simulink model "SWC_FDC_type"  (R2021b)
settings: Solver=FixedStepDiscrete  StartTime=0.0  StopTime=10.0  FixedStep=0.001  RelTol=1e-3
values from neighbouring files (symbols this model uses):
  C_TASK_5MS_S = (	C_TICK_TIME_S      	)    [vcu_local_hdr.m]
  DID_VCUKey = uint16(0x0202)    [vcu_local_hdr.m]
  DID_XWD = uint16(513)    [vcu_local_hdr.m]
  DIDLen_APPPedalZP = uint16(3)    [vcu_local_hdr.m]
  DIDLen_APSFunConfig = uint16(16)    [vcu_local_hdr.m]
  DIDLen_AutoLock = uint16(1)    [vcu_local_hdr.m]
  DIDLen_AutoWipHSpdEN = uint16(1)    [vcu_local_hdr.m]
  DIDLen_DKCKey = uint16(8)    [vcu_local_hdr.m]
  DIDLen_DRLDis = uint16(1)    [vcu_local_hdr.m]
  DIDLen_DynoMode = uint16(1)    [vcu_local_hdr.m]
  DIDLen_FMHTimer = uint16(1)    [vcu_local_hdr.m]
  DIDLen_LFLowPresThre = uint16(1)    [vcu_local_hdr.m]
  DIDLen_LFSensorID = uint16(4)    [vcu_local_hdr.m]
  DIDLen_LRLowPresThre = uint16(1)    [vcu_local_hdr.m]
  DIDLen_LRSensorID = uint16(4)    [vcu_local_hdr.m]
  DIDLen_NVMPedalZP = uint16(3)    [vcu_local_hdr.m]
  DIDLen_RFLowPresThre = uint16(1)    [vcu_local_hdr.m]
  DIDLen_RFSensorID = uint16(4)    [vcu_local_hdr.m]
  DIDLen_RRLowPresThre = uint16(1)    [vcu_local_hdr.m]
  DIDLen_RRSensorID = uint16(4)    [vcu_local_hdr.m]
  DIDLen_SensorMode = uint16(1)    [vcu_local_hdr.m]
  DIDLen_TireSize = uint16(16)    [vcu_local_hdr.m]
  DIDLen_TPMSLearnSta = uint16(1)    [vcu_local_hdr.m]
  DIDLen_TurnLampFLThreCurr = uint16(1)    [vcu_local_hdr.m]
  DIDLen_TurnLampFRThreCurr = uint16(1)    [vcu_local_hdr.m]
  DIDLen_TurnLampRLThreCurr = uint16(1)    [vcu_local_hdr.m]
  DIDLen_TurnLampRRThreCurr = uint16(1)    [vcu_local_hdr.m]
  DIDLen_USSConfig = uint16(16)    [vcu_local_hdr.m]
  DIDLen_WhlPres = uint16(4)    [vcu_local_hdr.m]
  DIDLen_WhlSensorBattSta = uint16(1)    [vcu_local_hdr.m]
  DIDLen_WhlTmp = uint16(4)    [vcu_local_hdr.m]
  DIDLen_WipRLSCmdCutFilter = uint16(1)    [vcu_local_hdr.m]
  DIDLen_WipRLSCmdHoldFilter = uint16(1)    [vcu_local_hdr.m]
  DIDLen_XWDMode = uint16(1)    [vcu_local_hdr.m]
  DIDNum_APPPedalZP = uint16(0x0206)    [vcu_local_hdr.m]
  DIDNum_APSFunConfig = uint16(0x0903)    [vcu_local_hdr.m]
  DIDNum_AutoLock = uint16(0x0306)    [vcu_local_hdr.m]
  DIDNum_AutoWipHSpdEN = uint16(0x0308)    [vcu_local_hdr.m]
  DIDNum_DKCKey = uint16(0x0202)    [vcu_local_hdr.m]
  DIDNum_DRLDis = uint16(0x0307)    [vcu_local_hdr.m]
  DIDNum_DynoMode = uint16(0x0203)    [vcu_local_hdr.m]
  DIDNum_FMHTimer = uint16(0x0305)    [vcu_local_hdr.m]
  DIDNum_LFLowPresThre = uint16(0x0B08)    [vcu_local_hdr.m]
  DIDNum_LFSensorID = uint16(0x0B01)    [vcu_local_hdr.m]
  DIDNum_LRLowPresThre = uint16(0x0B0A)    [vcu_local_hdr.m]
  DIDNum_LRSensorID = uint16(0x0B03)    [vcu_local_hdr.m]
  DIDNum_NVMPedalZP = uint16(0x0207)    [vcu_local_hdr.m]
  DIDNum_RFLowPresThre = uint16(0x0B09)    [vcu_local_hdr.m]
  DIDNum_RFSensorID = uint16(0x0B02)    [vcu_local_hdr.m]
  DIDNum_RRLowPresThre = uint16(0x0B0B)    [vcu_local_hdr.m]
  DIDNum_RRSensorID = uint16(0x0B04)    [vcu_local_hdr.m]
  DIDNum_SensorMode = uint16(0x0B0C)    [vcu_local_hdr.m]
  DIDNum_TireSize = uint16(0x0902)    [vcu_local_hdr.m]
  DIDNum_TPMSLearnSta = uint16(0x0B0D)    [vcu_local_hdr.m]
  DIDNum_TurnLampFLThreCurr = uint16(0x0303)    [vcu_local_hdr.m]
  DIDNum_TurnLampFRThreCurr = uint16(0x0301)    [vcu_local_hdr.m]
  DIDNum_TurnLampRLThreCurr = uint16(0x0304)    [vcu_local_hdr.m]
  DIDNum_TurnLampRRThreCurr = uint16(0x0302)    [vcu_local_hdr.m]
  DIDNum_USSConfig = uint16(0x0901)    [vcu_local_hdr.m]
  DIDNum_WhlPres = uint16(0x0B05)    [vcu_local_hdr.m]
  DIDNum_WhlSensorBattSta = uint16(0x0B07)    [vcu_local_hdr.m]
  DIDNum_WhlTmp = uint16(0x0B06)    [vcu_local_hdr.m]
  DIDNum_WipRLSCmdCutFilter = uint16(0x030A)    [vcu_local_hdr.m]
  DIDNum_WipRLSCmdHoldFilter = uint16(0x0309)    [vcu_local_hdr.m]
  DIDNum_XWDMode = uint16(0x0201)    [vcu_local_hdr.m]
  DIDVCUKeyLength = uint16(8)    [vcu_local_hdr.m]
  DTC_10020B = Simulink.Parameter    [DTC_Constant_Definition.m]
  DTC_10020C = Simulink.Parameter    [DTC_Constant_Definition.m]
  DTC_10020D = Simulink.Parameter    [DTC_Constant_Definition.m]
  DTC_10020E = Simulink.Parameter    [DTC_Constant_Definition.m]
  DTC_100210 = Simulink.Parameter    [DTC_Constant_Definition.m]
  DTC_100211 = Simulink.Parameter    [DTC_Constant_Definition.m]
  DTC_100212 = Simulink.Parameter    [DTC_Constant_Definition.m]
  DTC_100213 = Simulink.Parameter    [DTC_Constant_Definition.m]
  DTC_100214 = Simulink.Parameter    [DTC_Constant_Definition.m]
  DTC_100215 = Simulink.Parameter    [DTC_Constant_Definition.m]
  DTC_100216 = Simulink.Parameter    [DTC_Constant_Definition.m]
  DTC_100217 = Simulink.Parameter    [DTC_Constant_Definition.m]
  DTC_100218 = Simulink.Parameter    [DTC_Constant_Definition.m]
  DTC_100219 = Simulink.Parameter    [DTC_Constant_Definition.m]
  DTC_10021A = Simulink.Parameter    [DTC_Constant_Definition.m]
  DTC_10021B = Simulink.Parameter    [DTC_Constant_Definition.m]
  DTC_10021C = Simulink.Parameter    [DTC_Constant_Definition.m]
  DTC_10021D = Simulink.Parameter    [DTC_Constant_Definition.m]
  DTC_10021E = Simulink.Parameter    [DTC_Constant_Definition.m]
  DTC_100220 = Simulink.Parameter    [DTC_Constant_Definition.m]
  DTC_100221 = Simulink.Parameter    [DTC_Constant_Definition.m]
  DTC_100223 = Simulink.Parameter    [DTC_Constant_Definition.m]
  DTC_100224 = Simulink.Parameter    [DTC_Constant_Definition.m]
  DTC_100225 = Simulink.Parameter    [DTC_Constant_Definition.m]
  DTC_100226 = Simulink.Parameter    [DTC_Constant_Definition.m]
  DTC_100227 = Simulink.Parameter    [DTC_Constant_Definition.m]
  DTC_100242 = Simulink.Parameter    [DTC_Constant_Definition.m]
  DTC_100243 = Simulink.Parameter    [DTC_Constant_Definition.m]
  DTC_100244 = Simulink.Parameter    [DTC_Constant_Definition.m]
  DTC_100247 = Simulink.Parameter    [DTC_Constant_Definition.m]
  DTC_100248 = Simulink.Parameter    [DTC_Constant_Definition.m]
  DTC_100249 = Simulink.Parameter    [DTC_Constant_Definition.m]
  DTC_100250 = Simulink.Parameter    [DTC_Constant_Definition.m]
  DTC_100251 = Simulink.Parameter    [DTC_Constant_Definition.m]
  DTC_100252 = Simulink.Parameter    [DTC_Constant_Definition.m]
  DTC_100A10 = Simulink.Parameter    [DTC_Constant_Definition.m]
  DTC_100A12 = Simulink.Parameter    [DTC_Constant_Definition.m]
  DTC_100A16 = Simulink.Parameter    [DTC_Constant_Definition.m]
  DTC_100A17 = Simulink.Parameter    [DTC_Constant_Definition.m]
  DTC_100A18 = Simulink.Parameter    [DTC_Constant_Definition.m]
  DTC_100A19 = Simulink.Parameter    [DTC_Constant_Definition.m]
  DTC_500B01 = Simulink.Parameter    [DTC_Constant_Definition.m]
  DTC_500B02 = Simulink.Parameter    [DTC_Constant_Definition.m]
  DTC_500B03 = Simulink.Parameter    [DTC_Constant_Definition.m]
  DTC_500B04 = Simulink.Parameter    [DTC_Constant_Definition.m]
  DTC_500B05 = Simulink.Parameter    [DTC_Constant_Definition.m]
  DTC_500B06 = Simulink.Parameter    [DTC_Constant_Definition.m]
  DTC_500B07 = Simulink.Parameter    [DTC_Constant_Definition.m]
  DTC_500B08 = Simulink.Parameter    [DTC_Constant_Definition.m]
  DTC_500B09 = Simulink.Parameter    [DTC_Constant_Definition.m]
  DTC_500B0A = Simulink.Parameter    [DTC_Constant_Definition.m]
  DTC_500B0B = Simulink.Parameter    [DTC_Constant_Definition.m]
  DTC_500B0C = Simulink.Parameter    [DTC_Constant_Definition.m]
  DTC_500B0D = Simulink.Parameter    [DTC_Constant_Definition.m]
  ... (+93 more)
undefined symbols (not defined in the file or in its folder): f32_ApsOutVehSpdSig, KHAL_CANBusOffDebounce_cnt, KHAL_CANBusOffDebounce_s, KHAL_DKCDecryptEnable_flg_ovrdflg, KHAL_DKCDecryptEnable_flg_ovrdval, KHAL_RandomNumberY1_enum, KHAL_RandomNumberY2_enum, KHAL_RandomNumberY_ovrdflg, KHAL_TPMSRESBUTT_flg_ovrdflg, KHAL_TPMSRESBUTT_flg_ovrdval, KINP_ReadVinCode_flg, KTQD_DefaultRegenMode_enum, R_DIDWriteCDD_CSOP_DIDSet_APPPedalZP, R_DIDWriteCDD_CSOP_DIDSet_APSFunConfig, R_DIDWriteCDD_CSOP_DIDSet_AutoLock, R_DIDWriteCDD_CSOP_DIDSet_AutoWipHSpdEN, R_DIDWriteCDD_CSOP_DIDSet_DKCKey, R_DIDWriteCDD_CSOP_DIDSet_DRLDis, R_DIDWriteCDD_CSOP_DIDSet_DynoMode, R_DIDWriteCDD_CSOP_DIDSet_FMHTimer, R_DIDWriteCDD_CSOP_DIDSet_LFLowPresThre, R_DIDWriteCDD_CSOP_DIDSet_LFSensorID, R_DIDWriteCDD_CSOP_DIDSet_LRLowPresThre, R_DIDWriteCDD_CSOP_DIDSet_LRSensorID, R_DIDWriteCDD_CSOP_DIDSet_NVMPedalZP, R_DIDWriteCDD_CSOP_DIDSet_RFLowPresThre, R_DIDWriteCDD_CSOP_DIDSet_RFSensorID, R_DIDWriteCDD_CSOP_DIDSet_RRLowPresThre, R_DIDWriteCDD_CSOP_DIDSet_RRSensorID, R_DIDWriteCDD_CSOP_DIDSet_SensorMode, R_DIDWriteCDD_CSOP_DIDSet_TireSize, R_DIDWriteCDD_CSOP_DIDSet_TPMSLearnSta, R_DIDWriteCDD_CSOP_DIDSet_TurnLampFLThreCurr, R_DIDWriteCDD_CSOP_DIDSet_TurnLampFRThreCurr, R_DIDWriteCDD_CSOP_DIDSet_TurnLampRLThreCurr, R_DIDWriteCDD_CSOP_DIDSet_TurnLampRRThreCurr, R_DIDWriteCDD_CSOP_DIDSet_USSConfig, R_DIDWriteCDD_CSOP_DIDSet_WhlPres, R_DIDWriteCDD_CSOP_DIDSet_WhlSensorBattSta, R_DIDWriteCDD_CSOP_DIDSet_WhlTmp, R_DIDWriteCDD_CSOP_DIDSet_WipRLSCmdCutFilter, R_DIDWriteCDD_CSOP_DIDSet_WipRLSCmdHoldFilter, R_DIDWriteCDD_CSOP_DIDSet_XWDMode, R_E2E_CAN3_VCU1_CSOP_Write_CAN3_VCU1, R_E2E_CAN3_VCU1_toNIDEC_CSOP_Write_CAN3_VCU1_toNIDEC ... (+128)
libraries: simulink x246, FVT_lib x139, hcu_lib x31, hdlsllib x11, app x1, halin x1, halout x1, matrix_library x1, inp x1, outp x1
(part 5 of 13)

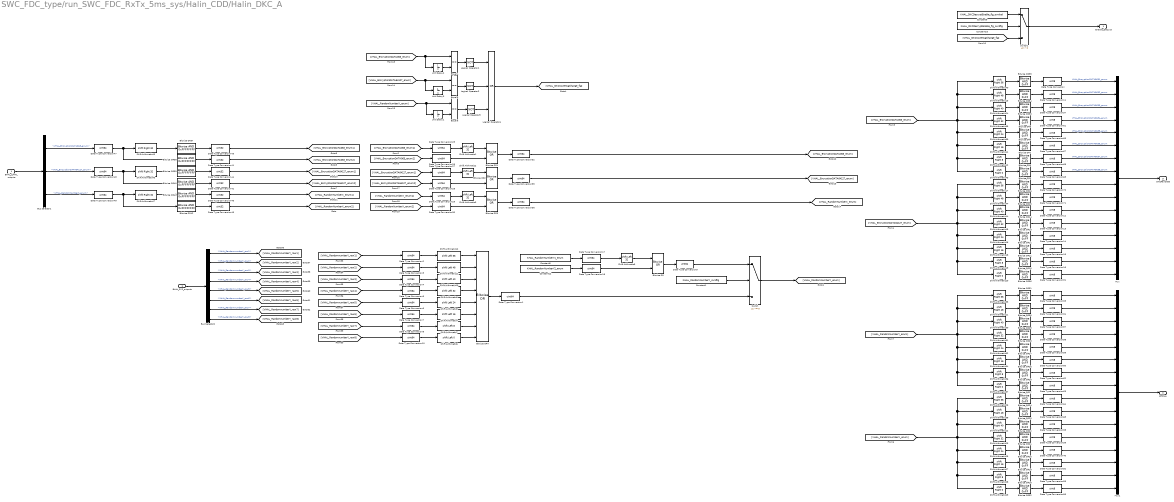
== system SWC_FDC_type/run_SWC_FDC_RxTx_5ms_sys/Halin_CDD/Halin_DKC_A ==
  BHAL_CAN4_outputs : Inport
  BHAL_SYS_outputs : Inport  Port=2
  Bitwise OR{,1..3} (4 alike) : simulink/Logic and Bit Operations/Bitwise Operator  logicop=OR  UseBitMask=off  NumInputPorts=2  BitMask=bin2dec('11011001')  BitMaskRealWorld=Stored Integer
  Bitwise OR{5..36} (32 alike) : simulink/Logic and Bit Operations/Bitwise Operator  logicop=AND  UseBitMask=on  BitMask=0xFF  BitMaskRealWorld=Stored Integer
  Bitwise OR{37..42} (6 alike) : simulink/Logic and Bit Operations/Bitwise Operator  logicop=AND  UseBitMask=on  BitMask=0xFFFFFFFF  BitMaskRealWorld=Stored Integer
  Bitwise OR4 : simulink/Logic and Bit Operations/Bitwise Operator  logicop=OR  UseBitMask=off  NumInputPorts=8  BitMask=bin2dec('11011001')  BitMaskRealWorld=Stored Integer
  Bus Selector1 : BusSelector  OutputSignals=VHAL_EncryptionDATA063_enum,VHAL_EncryptionDATA64127_enum,VHAL_RandomNumberX_enum
  Bus Selector2 : BusSelector  OutputSignals=VHAL_RandomnumberY_raw1,VHAL_RandomnumberY_raw2,VHAL_RandomnumberY_raw3,VHAL_RandomnumberY_raw4,VHAL_RandomnumberY_raw5,VHAL_RandomnumberY_raw6,VHAL_RandomnumberY_raw7,VHAL_RandomnumberY_raw8
  Constant1 : Constant  Value=KHAL_RandomNumberY_ovrdflg  OutDataTypeStr=uint64
  Constant10 : Constant  Value=KHAL_DKCDecryptEnable_flg_ovrdflg
  Constant12 : Constant  Value=KHAL_RandomNumberY2_enum  OutDataTypeStr=uint64
  Constant5 : Constant  Value=KHAL_RandomNumberY1_enum  OutDataTypeStr=uint64
  Constant9 : Constant  Value=KHAL_DKCDecryptEnable_flg_ovrdval
  Data Type Conversion{,11..16,31,33..34,37..40,52,55..71} (32 alike) : DataTypeConversion  OutDataTypeStr=uint8
  Data Type Conversion{1..10,17..18,25..30,32,35..36,47..49} (24 alike) : DataTypeConversion  OutDataTypeStr=uint64
  Data Type Conversion{41..46} (6 alike) : DataTypeConversion  OutDataTypeStr=uint32
  Equal4 : RelationalOperator  Operator===  OutDataTypeStr=boolean  RndMeth=Simplest
  Equal5 : RelationalOperator  Operator===  OutDataTypeStr=boolean  RndMeth=Simplest
  Equal6 : RelationalOperator  Operator===  OutDataTypeStr=boolean  RndMeth=Simplest
  Logical Operator1 : Logic  Operator=NOT  AllPortsSameDT=off  OutDataTypeStr=boolean
  Logical Operator2 : Logic  Operator=NOT  AllPortsSameDT=off  OutDataTypeStr=boolean
  Logical Operator3 : Logic  Operator=NOT  AllPortsSameDT=off  OutDataTypeStr=boolean
  Logical Operator4 : Logic  Operator=OR  Inputs=3  AllPortsSameDT=off  OutDataTypeStr=boolean
  Mux : Mux  Inputs=16
  Mux1 : Mux  Inputs=16
  Shift Arithmetic{1..3,5,9} (5 alike) : ArithShift  BitShiftNumber=32  BitShiftDirection=Left
  Shift Arithmetic10 : ArithShift  BitShiftNumber=40  BitShiftDirection=Left
  Shift Arithmetic11 : ArithShift  BitShiftNumber=48  BitShiftDirection=Left
  Shift Arithmetic12 : ArithShift  BitShiftNumber=56  BitShiftDirection=Left
  Shift Arithmetic{13,21,38,44} (4 alike) : ArithShift  BitShiftNumber=48  BitShiftDirection=Right
  Shift Arithmetic{14,22,24,30} (4 alike) : ArithShift  BitShiftNumber=40  BitShiftDirection=Right
  Shift Arithmetic{15,23,31,35,45..47} (7 alike) : ArithShift  BitShiftNumber=32  BitShiftDirection=Right
  Shift Arithmetic{16,25,32,39} (4 alike) : ArithShift  BitShiftNumber=24  BitShiftDirection=Right
  Shift Arithmetic{17,26,33,40} (4 alike) : ArithShift  BitShiftNumber=56  BitShiftDirection=Right
  Shift Arithmetic{18,27,34,41} (4 alike) : ArithShift  BitShiftNumber=16  BitShiftDirection=Right
  Shift Arithmetic{19,28,36,42} (4 alike) : ArithShift  BitShiftNumber=8  BitShiftDirection=Right
  Shift Arithmetic{20,29,37,43} (4 alike) : ArithShift  BitShiftDirection=Right
  Shift Arithmetic4 : ArithShift  BitShiftNumber=16  BitShiftDirection=Left
  Shift Arithmetic6 : ArithShift  BitShiftDirection=Left
  Shift Arithmetic7 : ArithShift  BitShiftNumber=8  BitShiftDirection=Left
  Shift Arithmetic8 : ArithShift  BitShiftNumber=24  BitShiftDirection=Left
  Switch : Switch  Criteria=u2 ~= 0
  Switch1 : Switch  Criteria=u2 > Threshold
  Unit Delay1 : UnitDelay  SampleTime=-1  HasFrameUpgradeWarning=on
  Unit Delay2 : UnitDelay  SampleTime=-1  HasFrameUpgradeWarning=on
  Unit Delay3 : UnitDelay  SampleTime=-1  HasFrameUpgradeWarning=on
  Enable_Decrypt : Outport
  AESKey : Outport  Port=2
  DKCRawData : Outport  Port=3
  wires:
  Data Type Conversion8/1 -> Shift Arithmetic7/1
  Bitwise OR5/1 -> Data Type Conversion69/1
  [VHAL_RandomNumberX_enum] -> Shift Arithmetic38/1, Shift Arithmetic26/1, Shift Arithmetic22/1, Shift Arithmetic25/1, Shift Arithmetic27/1, Shift Arithmetic29/1, Shift Arithmetic28/1, Shift Arithmetic23/1
  Shift Arithmetic17/1 -> Bitwise OR16/1
  Data Type Conversion52/1 -> Mux1/14
  Bitwise OR35/1 -> Data Type Conversion/1
  Shift Arithmetic13/1 -> Bitwise OR34/1
  Data Type Conversion42/1 -> [VHAL_EncryptionDATA64127_enum2]
  Bitwise OR/1 -> Data Type Conversion9/1
  [VHAL_EncryptionDATA64127_enum] -> Shift Arithmetic15/1, Shift Arithmetic19/1, Shift Arithmetic20/1, Shift Arithmetic18/1, Shift Arithmetic16/1, Shift Arithmetic14/1, Shift Arithmetic17/1, Shift Arithmetic44/1
  [VHAL_RandomnumberY_raw5] -> Data Type Conversion6/1
  Shift Arithmetic7/1 -> Bitwise OR4/7
  [VHAL_RandomnumberY_raw4] -> Data Type Conversion5/1
  [VHAL_RandomNumberX_enum] -> Equal6/1, Unit Delay1/1
  [VHAL_EncryptionDATA063_enum] -> Shift Arithmetic13/1, Shift Arithmetic40/1, Shift Arithmetic24/1, Shift Arithmetic39/1, Shift Arithmetic41/1, Shift Arithmetic43/1, Shift Arithmetic42/1, Shift Arithmetic35/1
  Bus Selector2/3 -> [VHAL_RandomnumberY_raw3]  "<VHAL_RandomnumberY_raw3>"
  Bitwise OR15/1 -> Data Type Conversion71/1
  Bus Selector2/2 -> [VHAL_RandomnumberY_raw2]  "<VHAL_RandomnumberY_raw2>"
  [VHAL_RandomnumberY_raw1] -> Data Type Conversion2/1
  Data Type Conversion69/1 -> Mux/8  "VHAL_EncryptionDATA0638_enum"
  Data Type Conversion37/1 -> Mux/3  "VHAL_EncryptionDATA0633_enum"
  Data Type Conversion5/1 -> Shift Arithmetic9/1
  Bitwise OR8/1 -> Data Type Conversion66/1
  Bitwise OR14/1 -> Data Type Conversion12/1
  Bus Selector2/1 -> [VHAL_RandomnumberY_raw1]  "<VHAL_RandomnumberY_raw1>"
  Bitwise OR17/1 -> Data Type Conversion63/1
  Data Type Conversion34/1 -> Mux1/2
  Bus Selector2/5 -> [VHAL_RandomnumberY_raw5]  "<VHAL_RandomnumberY_raw5>"
  Shift Arithmetic35/1 -> Bitwise OR9/1
  Data Type Conversion67/1 -> Mux/6  "VHAL_EncryptionDATA0636_enum"
  Bus Selector2/6 -> [VHAL_RandomnumberY_raw6]  "<VHAL_RandomnumberY_raw6>"
  Data Type Conversion9/1 -> Switch/1
  Data Type Conversion10/1 -> Shift Arithmetic6/1
  Data Type Conversion45/1 -> [VHAL_RandomNumberX_enum2]
  Data Type Conversion13/1 -> Mux/12
  Data Type Conversion1/1 -> Switch/3
  [VHAL_RandomnumberY_raw2] -> Data Type Conversion3/1
  BHAL_SYS_outputs/1 -> Bus Selector2/1
  Shift Arithmetic25/1 -> Bitwise OR20/1
  [VHAL_EncryptionDATA063_enum1] -> Data Type Conversion25/1
  Logical Operator3/1 -> Logical Operator4/3
  Shift Arithmetic6/1 -> Bitwise OR4/8
  Data Type Conversion70/1 -> Mux/9
  Data Type Conversion66/1 -> Mux/5  "VHAL_EncryptionDATA0635_enum"
  [VHAL_EncryptionDATA64127_enum] -> Equal5/1, Unit Delay3/1
  Data Type Conversion14/1 -> Mux/13
  Shift Arithmetic10/1 -> Bitwise OR4/3
  Data Type Conversion40/1 -> Mux1/13
  Unit Delay1/1 -> Equal6/2
  Data Type Conversion43/1 -> [VHAL_EncryptionDATA063_enum1]
  Unit Delay3/1 -> Equal5/2
  Bitwise OR31/1 -> Data Type Conversion33/1
  Shift Arithmetic12/1 -> Bitwise OR4/1
  [VHAL_RandomnumberY_raw3] -> Data Type Conversion4/1
  Shift Arithmetic28/1 -> Bitwise OR18/1
  Constant1/1 -> Switch/2
  Data Type Conversion7/1 -> Shift Arithmetic4/1
  Bitwise OR4/1 -> Data Type Conversion1/1
  Bitwise OR21/1 -> Data Type Conversion39/1
  Shift Arithmetic11/1 -> Bitwise OR4/2
  Data Type Conversion31/1 -> Mux/16
  Shift Arithmetic2/1 -> Bitwise OR2/1
  Data Type Conversion68/1 -> Mux/7  "VHAL_EncryptionDATA0637_enum"
  Data Type Conversion4/1 -> Shift Arithmetic10/1
  Bus Selector2/7 -> [VHAL_RandomnumberY_raw7]  "<VHAL_RandomnumberY_raw7>"
  Data Type Conversion12/1 -> Mux/11
  Data Type Conversion30/1 -> Bitwise OR3/2
  Data Type Conversion32/1 -> [VHAL_EncryptionDATA063_enum]
  [VHAL_RandomNumberY_enum] -> Shift Arithmetic31/1, Shift Arithmetic36/1, Shift Arithmetic37/1, Shift Arithmetic34/1, Shift Arithmetic32/1, Shift Arithmetic30/1, Shift Arithmetic33/1, Shift Arithmetic21/1
  Shift Arithmetic14/1 -> Bitwise OR14/1
  Data Type Conversion55/1 -> Mux1/15
  Shift Arithmetic33/1 -> Bitwise OR31/1
  Data Type Conversion59/1 -> Mux1/5
  Shift Arithmetic21/1 -> Bitwise OR30/1
  Shift Arithmetic18/1 -> Bitwise OR11/1
  [VHAL_EncryptionDATA64127_enum2] -> Data Type Conversion28/1
  [VHAL_RandomNumberX_enum2] -> Data Type Conversion30/1
  Shift Arithmetic1/1 -> Bitwise OR1/1
  Data Type Conversion18/1 -> Bitwise OR/2
  Shift Arithmetic26/1 -> Bitwise OR24/1
  Shift Arithmetic15/1 -> Bitwise OR13/1
  Shift Arithmetic23/1 -> Bitwise OR21/1
  Data Type Conversion39/1 -> Mux1/12
  Bitwise OR2/1 -> Data Type Conversion35/1
  Bitwise OR25/1 -> Data Type Conversion62/1
  Bitwise OR36/1 -> Data Type Conversion31/1
  Data Type Conversion15/1 -> Mux/14
  Bitwise OR11/1 -> Data Type Conversion15/1
  Switch/1 -> [VHAL_RandomNumberY_enum]
  Shift Arithmetic9/1 -> Bitwise OR4/4
  Bitwise OR7/1 -> Data Type Conversion67/1
  Data Type Conversion35/1 -> [VHAL_EncryptionDATA64127_enum]
  Shift Arithmetic29/1 -> Bitwise OR32/1
  Data Type Conversion58/1 -> Mux1/4
  Bitwise OR1/1 -> Data Type Conversion32/1
  Bitwise OR27/1 -> Data Type Conversion59/1
  Data Type Conversion33/1 -> Mux1/1
  Bitwise OR24/1 -> Data Type Conversion64/1
  Bitwise OR22/1 -> Data Type Conversion38/1
  Data Type Conversion/1 -> Mux/1  "VHAL_EncryptionDATA0631_enum"
  Equal5/1 -> Logical Operator2/1
  [VHAL_EncryptionDATA063_enum2] -> Data Type Conversion26/1
  [VHAL_RandomnumberY_raw8] -> Data Type Conversion10/1
  [VHAL_EncryptionDATA063_enum] -> Equal4/1, Unit Delay2/1
  Data Type Conversion36/1 -> [VHAL_RandomNumberX_enum]
  Data Type Conversion29/1 -> Shift Arithmetic3/1
  Shift Arithmetic8/1 -> Bitwise OR4/5
  Bitwise OR29/1 -> Data Type Conversion57/1
  Data Type Conversion28/1 -> Bitwise OR2/2
  Constant12/1 -> Data Type Conversion18/1
  Data Type Conversion26/1 -> Bitwise OR1/2
  Shift Arithmetic31/1 -> Bitwise OR28/1
  Data Type Conversion25/1 -> Shift Arithmetic1/1
  Logical Operator2/1 -> Logical Operator4/2
  [VHAL_RandomNumberX_enum1] -> Data Type Conversion29/1
  Constant5/1 -> Data Type Conversion17/1
  Bitwise OR23/1 -> Data Type Conversion65/1
  Shift Arithmetic4/1 -> Bitwise OR4/6
  Data Type Conversion41/1 -> [VHAL_EncryptionDATA063_enum2]
  Data Type Conversion2/1 -> Shift Arithmetic12/1
  Shift Arithmetic24/1 -> Bitwise OR33/1
  Shift Arithmetic3/1 -> Bitwise OR3/1
  [VHAL_RandomnumberY_raw7] -> Data Type Conversion8/1
  Bus Selector2/8 -> [VHAL_RandomnumberY_raw8]  "<VHAL_RandomnumberY_raw8>"
  Shift Arithmetic41/1 -> Bitwise OR7/1
  [VHAL_EncryptionDATA64127_enum1] -> Data Type Conversion27/1
  [VHAL_RandomnumberY_raw6] -> Data Type Conversion7/1
  Bitwise OR3/1 -> Data Type Conversion36/1
  Data Type Conversion17/1 -> Shift Arithmetic5/1
  Logical Operator4/1 -> [VHAL_DKCCANMsgChange_flg]
  Data Type Conversion44/1 -> [VHAL_EncryptionDATA64127_enum1]
  Data Type Conversion11/1 -> Mux/2  "VHAL_EncryptionDATA0632_enum"
  Data Type Conversion3/1 -> Shift Arithmetic11/1
  Shift Arithmetic36/1 -> Bitwise OR25/1
  Data Type Conversion27/1 -> Shift Arithmetic2/1
  Unit Delay2/1 -> Equal4/2
  Equal6/1 -> Logical Operator3/1
  Bus Selector2/4 -> [VHAL_RandomnumberY_raw4]  "<VHAL_RandomnumberY_raw4>"
  Shift Arithmetic5/1 -> Bitwise OR/1
  Data Type Conversion6/1 -> Shift Arithmetic8/1
  Equal4/1 -> Logical Operator1/1
  Data Type Conversion46/1 -> [VHAL_RandomNumberX_enum1]
  Data Type Conversion71/1 -> Mux/10
  Logical Operator1/1 -> Logical Operator4/1
  Shift Arithmetic44/1 -> Bitwise OR15/1
  Shift Arithmetic43/1 -> Bitwise OR5/1
  Shift Arithmetic27/1 -> Bitwise OR19/1
  Shift Arithmetic34/1 -> Bitwise OR26/1
  Bitwise OR9/1 -> Data Type Conversion61/1
  Data Type Conversion62/1 -> Mux1/7
  Shift Arithmetic16/1 -> Bitwise OR12/1
  Shift Arithmetic19/1 -> Bitwise OR10/1
  Mux/1 -> DKCRawData/1
  Bitwise OR6/1 -> Data Type Conversion68/1
  Shift Arithmetic40/1 -> Bitwise OR35/1
  Bitwise OR26/1 -> Data Type Conversion60/1
  Bitwise OR12/1 -> Data Type Conversion14/1
  Data Type Conversion63/1 -> Mux1/8
  Data Type Conversion65/1 -> Mux1/10
  Shift Arithmetic42/1 -> Bitwise OR6/1
  Bitwise OR16/1 -> Data Type Conversion70/1
  Bitwise OR33/1 -> Data Type Conversion37/1
  Shift Arithmetic22/1 -> Bitwise OR22/1
  Bitwise OR32/1 -> Data Type Conversion56/1
  Data Type Conversion38/1 -> Mux1/11
  Shift Arithmetic39/1 -> Bitwise OR8/1
  Bitwise OR10/1 -> Data Type Conversion16/1
  Data Type Conversion16/1 -> Mux/15
  Data Type Conversion56/1 -> Mux1/16
  Shift Arithmetic20/1 -> Bitwise OR36/1
  Bitwise OR13/1 -> Data Type Conversion13/1
  Bitwise OR19/1 -> Data Type Conversion52/1
  Bitwise OR18/1 -> Data Type Conversion55/1
  Data Type Conversion64/1 -> Mux1/9
  Data Type Conversion61/1 -> Mux/4  "VHAL_EncryptionDATA0634_enum"
  Shift Arithmetic32/1 -> Bitwise OR27/1
  Data Type Conversion60/1 -> Mux1/6
  Bitwise OR28/1 -> Data Type Conversion58/1
  Shift Arithmetic38/1 -> Bitwise OR23/1
  Bitwise OR20/1 -> Data Type Conversion40/1
  Shift Arithmetic30/1 -> Bitwise OR29/1
  Bitwise OR34/1 -> Data Type Conversion11/1
  Shift Arithmetic37/1 -> Bitwise OR17/1
  Data Type Conversion57/1 -> Mux1/3
  Bitwise OR30/1 -> Data Type Conversion34/1
  Mux1/1 -> AESKey/1
  Constant9/1 -> Switch1/1
  [VHAL_DKCCANMsgChange_flg] -> Switch1/3
  Constant10/1 -> Switch1/2
  Switch1/1 -> Enable_Decrypt/1
  Bitwise OR42/1 -> Data Type Conversion45/1
  Bitwise OR40/1 -> Data Type Conversion42/1
  Bus Selector1/1 -> Data Type Conversion47/1  "<VHAL_EncryptionDATA063_enum>"
  Shift Arithmetic46/1 -> Bitwise OR39/1
  Bitwise OR38/1 -> Data Type Conversion41/1
  Data Type Conversion49/1 -> Bitwise OR42/1, Shift Arithmetic47/1
  Bitwise OR41/1 -> Data Type Conversion46/1
  Data Type Conversion48/1 -> Bitwise OR40/1, Shift Arithmetic46/1
  Shift Arithmetic47/1 -> Bitwise OR41/1
  Shift Arithmetic45/1 -> Bitwise OR37/1
  Data Type Conversion47/1 -> Bitwise OR38/1, Shift Arithmetic45/1
  Bus Selector1/2 -> Data Type Conversion48/1  "<VHAL_EncryptionDATA64127_enum>"
  Bitwise OR39/1 -> Data Type Conversion44/1
  Bitwise OR37/1 -> Data Type Conversion43/1
  Bus Selector1/3 -> Data Type Conversion49/1  "<VHAL_RandomNumberX_enum>"
  BHAL_CAN4_outputs/1 -> Bus Selector1/1

== system SWC_FDC_type/run_SWC_FDC_RxTx_5ms_sys/Halin_CDD/Halin_GPIO ==
  VHAL_AccelPedal1Vol_Raw : Inport
  VHAL_AccelPedal2Vol_Raw : Inport  Port=2
  VHAL_BrakeSWGPIO_flg : Inport  Port=3
  VHAL_HoodSW_flg : Inport  Port=4
  VHAL_TailgateSW_flg : Inport  Port=5
  VHAL_DrDoorSW_flg : Inport  Port=6
  VHAL_PsDoorSW_flg : Inport  Port=7
  VHAL_RRDoorSW_flg : Inport  Port=8
  VHAL_RLDoorSW_flg : Inport  Port=9
  VHAL_CentralDoorLockSW_flg : Inport  Port=10
  VHAL_HazardSW_flg : Inport  Port=11
  VHAL_BrakeLampSW_flg : Inport  Port=12
  VHAL_TrunkHanSW_flg : Inport  Port=13
  VHAL_SeatSW_flg : Inport  Port=14
  VHAL_CrashSignalGPIO_flg : Inport  Port=15
  u8_HWID_4byte : Inport  Port=16
  u8_GetHWIDSta : Inport  Port=17
  Bus Creator : BusCreator  Inputs=21
  Data Type Conversion{1,3..4,17} (4 alike) : DataTypeConversion  OutDataTypeStr=single
  Data Type Conversion{2,5..10,12..16,18,22} (14 alike) : DataTypeConversion  OutDataTypeStr=boolean
  Data Type Conversion{11,19..21} (4 alike) : DataTypeConversion  OutDataTypeStr=uint8
  Demux1 : Demux  Commented=on
  Demux2 : Demux
  From : From  Commented=on  GotoTag=VHAL_GetHWIDErr_flg
  From1 : From  Commented=on  GotoTag=u8_HWID_4byte
  Gain : Gain  Gain=5/4095
  Gain1 : Gain  Gain=5/4095
  Goto2 : Goto  Commented=on  GotoTag=VHAL_HWID2_enum
  Goto4 : Goto  Commented=on  GotoTag=VHAL_HWID3_enum
  Goto5 : Goto  Commented=on  GotoTag=VHAL_HWID4_enum
  Goto7 : Goto  Commented=on  GotoTag=VHAL_HWID1_enum
  Ground3 : Ground
  Ground4 : Ground
  Logical Operator{2..13} (12 alike) : Logic  Operator=NOT  AllPortsSameDT=off  OutDataTypeStr=boolean
  String Constant : StringConstant  Commented=on  String="\"----\""
  String to ASCII : StringToASCII  Commented=on  OutputVectorSize=4
  Switch : Switch  Commented=on  Criteria=u2 > Threshold
  Transpose : matrix_library/Transpose  Commented=on
      settings: SourceProductBaseCode=SL
  BHAL_GPIO_outputs : Outport
  wires:
  Data Type Conversion7/1 -> Bus Creator/7  "VHAL_TailgateSW_flg"
  Data Type Conversion9/1 -> Bus Creator/9  "VHAL_PsDoorSW_flg"
  Logical Operator6/1 -> Data Type Conversion9/1
  Gain1/1 -> Bus Creator/2  "VHAL_AccelPedal2Vol_V"
  Logical Operator3/1 -> Data Type Conversion7/1
  Data Type Conversion15/1 -> Bus Creator/16  "VHAL_SeatSW_flg"
  Data Type Conversion4/1 -> Bus Creator/4  "VHAL_CrashInputDuty_pct"
  Data Type Conversion10/1 -> Bus Creator/11  "VHAL_RLDoorSW_flg"
  Logical Operator5/1 -> Data Type Conversion8/1
  Data Type Conversion1/1 -> Gain/1
  VHAL_PsDoorSW_flg/1 -> Logical Operator6/1
  VHAL_AccelPedal1Vol_Raw/1 -> Data Type Conversion1/1
  Data Type Conversion18/1 -> Bus Creator/10  "VHAL_RRDoorSW_flg"
  VHAL_DrDoorSW_flg/1 -> Logical Operator5/1
  Logical Operator11/1 -> Data Type Conversion13/1
  Logical Operator9/1 -> Data Type Conversion2/1
  Logical Operator4/1 -> Data Type Conversion6/1
  VHAL_RLDoorSW_flg/1 -> Logical Operator8/1
  Logical Operator12/1 -> Data Type Conversion14/1
  Data Type Conversion8/1 -> Bus Creator/8  "VHAL_DrDoorSW_flg"
  Gain/1 -> Bus Creator/1  "VHAL_AccelPedal1Vol_V"
  VHAL_HoodSW_flg/1 -> Logical Operator4/1
  Logical Operator10/1 -> Data Type Conversion12/1
  Data Type Conversion14/1 -> Bus Creator/15  "VHAL_TrunkHanSW_flg"
  Data Type Conversion13/1 -> Bus Creator/14  "VHAL_BrakeLampSW_flg"
  Logical Operator7/1 -> Data Type Conversion18/1
  Data Type Conversion17/1 -> Gain1/1
  Logical Operator13/1 -> Data Type Conversion15/1
  Data Type Conversion5/1 -> Bus Creator/5  "VHAL_BrakeSWGPIO_flg"
  Data Type Conversion2/1 -> Bus Creator/12  "VHAL_CentralDoorLockSW_flg"
  VHAL_CentralDoorLockSW_flg/1 -> Logical Operator9/1
  Logical Operator2/1 -> Data Type Conversion5/1
  Data Type Conversion6/1 -> Bus Creator/6  "VHAL_HoodSW_flg"
  Data Type Conversion16/1 -> Bus Creator/17  "VHAL_CrashSignalGPIO_flg"
  Ground4/1 -> Data Type Conversion4/1
  Data Type Conversion3/1 -> Bus Creator/3  "VHAL_CrashInputFreq_Hz"
  VHAL_BrakeLampSW_flg/1 -> Logical Operator11/1
  VHAL_AccelPedal2Vol_Raw/1 -> Data Type Conversion17/1
  VHAL_TailgateSW_flg/1 -> Logical Operator3/1
  Data Type Conversion12/1 -> Bus Creator/13  "VHAL_HazardSW_flg"
  Ground3/1 -> Data Type Conversion3/1
  VHAL_TrunkHanSW_flg/1 -> Logical Operator12/1
  VHAL_RRDoorSW_flg/1 -> Logical Operator7/1
  VHAL_HazardSW_flg/1 -> Logical Operator10/1
  Logical Operator8/1 -> Data Type Conversion10/1
  VHAL_CrashSignalGPIO_flg/1 -> Data Type Conversion16/1
  VHAL_SeatSW_flg/1 -> Logical Operator13/1
  VHAL_BrakeSWGPIO_flg/1 -> Logical Operator2/1
  Bus Creator/1 -> BHAL_GPIO_outputs/1
  [VHAL_HWID2_enum] -> Data Type Conversion19/1
  [VHAL_HWID3_enum] -> Data Type Conversion20/1
  Data Type Conversion11/1 -> Bus Creator/18  "VHAL_HWID1_enum"
  Data Type Conversion19/1 -> Bus Creator/19  "VHAL_HWID2_enum"
  Data Type Conversion20/1 -> Bus Creator/20  "VHAL_HWID3_enum"
  [VHAL_HWID4_enum] -> Data Type Conversion21/1
  Data Type Conversion21/1 -> Bus Creator/21  "VHAL_HWID4_enum"
  [VHAL_HWID1_enum] -> Data Type Conversion11/1
  Demux1/4 -> Goto5/1
  Demux1/3 -> Goto4/1
  Switch/1 -> Demux1/1
  String Constant/1 -> String to ASCII/1
  Transpose/1 -> Switch/1
  Demux1/1 -> Goto7/1
  Data Type Conversion22/1 -> [VHAL_GetHWIDErr_flg]
  u8_GetHWIDSta/1 -> Data Type Conversion22/1
  Demux1/2 -> Goto2/1
  String to ASCII/1 -> Transpose/1
  From/1 -> Switch/2
  From1/1 -> Switch/3
  u8_HWID_4byte/1 -> [u8_HWID_4byte]
  Demux2/2 -> [VHAL_HWID2_enum]
  Demux2/1 -> [VHAL_HWID1_enum]
  [u8_HWID_4byte] -> Demux2/1
  Demux2/3 -> [VHAL_HWID3_enum]
  Demux2/4 -> [VHAL_HWID4_enum]

== system SWC_FDC_type/run_SWC_FDC_RxTx_5ms_sys/Halin_CDD/Halin_IMU ==
  VHAL_IMUOffsetVal_raw : Inport
  VHAL_IMUSixAxisVal_raw : Inport  Port=2
  VHAL_IMUOffsetValSta_flg : Inport  Port=3
  VHAL_IMUSixAxisValSta_flg : Inport  Port=4
  Bus Creator : BusCreator  Inputs=12
  Constant{,1..4} (5 alike) : Constant  Value=0  OutDataTypeStr=int16
  Constant5 : Constant  Value=2000  OutDataTypeStr=int16
  Data Type Conversion{,1..11} (12 alike) : DataTypeConversion  OutDataTypeStr=int16
  Data Type Conversion12 : DataTypeConversion  OutDataTypeStr=boolean
  Data Type Conversion13 : DataTypeConversion  OutDataTypeStr=boolean
  Demux : Demux  Outputs=6
  Demux1 : Demux  Outputs=6
  Switch{,1..11} (12 alike) : Switch  Criteria=u2 ~= 0
  Unit Delay{6..11} (6 alike) : UnitDelay  SampleTime=-1  HasFrameUpgradeWarning=on
  BHAL_IMU_outputs : Outport
  wires:
  Demux1/2 -> Data Type Conversion7/1
  Bus Creator/1 -> BHAL_IMU_outputs/1
  Demux1/3 -> Data Type Conversion8/1
  Demux1/6 -> Data Type Conversion11/1
  Demux/1 -> Data Type Conversion/1
  Demux1/5 -> Data Type Conversion10/1
  Demux/6 -> Data Type Conversion5/1
  Demux/4 -> Data Type Conversion3/1
  Demux/5 -> Data Type Conversion4/1
  Demux1/4 -> Data Type Conversion9/1
  [VHAL_MemOffsetGyroX_raw16] -> Switch/3
  Demux1/1 -> Data Type Conversion6/1
  Demux/2 -> Data Type Conversion1/1
  Demux/3 -> Data Type Conversion2/1
  VHAL_IMUOffsetValSta_flg/1 -> Data Type Conversion12/1
  Switch/1 -> Bus Creator/1  "VHAL_MemOffsetGyroX_raw16"
  [VHAL_IMUOffsetValSta_flg] -> Switch/2
  Switch1/1 -> Bus Creator/2  "VHAL_MemOffsetGyroY_raw16"
  [VHAL_MemOffsetGyroY_raw16] -> Switch1/3
  [VHAL_MemOffsetGyroZ_raw16] -> Switch2/3
  Switch2/1 -> Bus Creator/3  "VHAL_MemOffsetGyroZ_raw16"
  Switch3/1 -> Bus Creator/4  "VHAL_MemOffsetAccX_raw16"
  [VHAL_MemOffsetAccX_raw16] -> Switch3/3
  [VHAL_MemOffsetAccY_raw16] -> Switch4/3
  Switch4/1 -> Bus Creator/5  "VHAL_MemOffsetAccY_raw16"
  Switch5/1 -> Bus Creator/6  "VHAL_MemOffsetAccZ_raw16"
  [VHAL_MemOffsetAccZ_raw16] -> Switch5/3
  [VHAL_SensingGyroX_raw16] -> Switch6/3
  Switch6/1 -> Bus Creator/7, Unit Delay6/1  "VHAL_SensingGyroX_raw16"
  Unit Delay6/1 -> Switch6/1
  Unit Delay7/1 -> Switch7/1
  Switch7/1 -> Bus Creator/8, Unit Delay7/1  "VHAL_SensingGyroY_raw16"
  [VHAL_SensingGyroY_raw16] -> Switch7/3
  [VHAL_SensingGyroZ_raw16] -> Switch8/3
  Switch8/1 -> Bus Creator/9, Unit Delay8/1  "VHAL_SensingGyroZ_raw16"
  Unit Delay8/1 -> Switch8/1
  Unit Delay9/1 -> Switch9/1
  Switch9/1 -> Bus Creator/10, Unit Delay9/1  "VHAL_SensingAccX_raw16"
  [VHAL_SensingAccX_raw16] -> Switch9/3
  [VHAL_SensingAccY_raw16] -> Switch10/3
  Switch10/1 -> Bus Creator/11, Unit Delay10/1  "VHAL_SensingAccY_raw16"
  Unit Delay10/1 -> Switch10/1
  Unit Delay11/1 -> Switch11/1
  Switch11/1 -> Bus Creator/12, Unit Delay11/1  "VHAL_SensingAccZ_raw16"
  [VHAL_SensingAccZ_raw16] -> Switch11/3
  Constant/1 -> Switch/1
  Constant1/1 -> Switch1/1
  [VHAL_IMUOffsetValSta_flg] -> Switch1/2
  Constant2/1 -> Switch2/1
  [VHAL_IMUOffsetValSta_flg] -> Switch2/2
  Constant3/1 -> Switch3/1
  [VHAL_IMUOffsetValSta_flg] -> Switch3/2
  Constant4/1 -> Switch4/1
  [VHAL_IMUOffsetValSta_flg] -> Switch4/2
  Constant5/1 -> Switch5/1
  [VHAL_IMUOffsetValSta_flg] -> Switch5/2
  [VHAL_IMUSixAxisValSta_flg] -> Switch6/2
  [VHAL_IMUSixAxisValSta_flg] -> Switch7/2
  [VHAL_IMUSixAxisValSta_flg] -> Switch8/2
  [VHAL_IMUSixAxisValSta_flg] -> Switch9/2
  [VHAL_IMUSixAxisValSta_flg] -> Switch10/2
  [VHAL_IMUSixAxisValSta_flg] -> Switch11/2
  VHAL_IMUOffsetVal_raw/1 -> Demux/1
  VHAL_IMUSixAxisVal_raw/1 -> Demux1/1
  Data Type Conversion/1 -> [VHAL_MemOffsetAccX_raw16]
  Data Type Conversion1/1 -> [VHAL_MemOffsetAccY_raw16]
  Data Type Conversion2/1 -> [VHAL_MemOffsetAccZ_raw16]
  Data Type Conversion3/1 -> [VHAL_MemOffsetGyroX_raw16]
  Data Type Conversion4/1 -> [VHAL_MemOffsetGyroY_raw16]
  Data Type Conversion5/1 -> [VHAL_MemOffsetGyroZ_raw16]
  Data Type Conversion6/1 -> [VHAL_SensingAccX_raw16]
  Data Type Conversion8/1 -> [VHAL_SensingAccZ_raw16]
  Data Type Conversion7/1 -> [VHAL_SensingAccY_raw16]
  Data Type Conversion10/1 -> [VHAL_SensingGyroY_raw16]
  Data Type Conversion9/1 -> [VHAL_SensingGyroX_raw16]
  Data Type Conversion11/1 -> [VHAL_SensingGyroZ_raw16]
  Data Type Conversion12/1 -> [VHAL_IMUOffsetValSta_flg]  "VHAL_IMUOffsetValSta_flg"
  Data Type Conversion13/1 -> [VHAL_IMUSixAxisValSta_flg]  "VHAL_IMUSixAxisValSta_flg"
  VHAL_IMUSixAxisValSta_flg/1 -> Data Type Conversion13/1
